simulink model "PLANTA_COMPLETA"  (R2024b)
settings: Solver=FixedStepAuto  StartTime=0.0  StopTime=inf  FixedStep=0.001  MaxStep=0.0005  RelTol=1e-4
undefined symbols (not defined in the file): A_hm, A_tm, at_breakpoints, at_max, b_ha, B_hm, b_ta, B_tm, bcx, bcy, bhd, bhEb, bhm, bt, btd, btm, btw, bwu, C_hm, C_tm, D_hm, D_tm, DiscIntNeverNeededParam, dl_h_ini, dx_l_ini, dx_t_ini, dx_td_ini, dxt_max, dy_l_ini, F01_a_t_max, F01_Ts1, F02_a_h_max, F02_Ts1, F03_a_h_max, F03_a_t_max, F03_dxt_max, F03_Ts1, Fhw_min, g, Hc, ih, it, Jhd_hEb, Jhm_hb, Jtd, Jtm_tb, K_hsa, K_hsia, K_tsa, K_tsia, Kcy, Kd_table, Ke_tita, Ke_w, kp_pos, Kp_table, kp_w, Ktw, kwu, l_breakpoints ... (+30)
libraries: simulink x13, spsEdgeDetectorLib x5, simulink_extras x2, dspsigops x2, vrlib x1, dspstat3 x1
(part 3 of 5)

== system PLANTA_COMPLETA/Masa contenedor ==
  Fwh : Inport
  TLK : Inport  Port=2
  Edge Detector : spsEdgeDetectorLib/Edge Detector  model=Falling  ic=0  Ts=-1
      settings: LibrarySourceBlock=sps_lib/Control/Edge Detector
  Edge Detector1 : spsEdgeDetectorLib/Edge Detector  model=Rising  ic=0  Ts=-1
      settings: LibrarySourceBlock=sps_lib/Control/Edge Detector
  Gain8 : Gain  Gain=2/g
  Product : Product
  S-R Flip-Flop : simulink_extras/Flip Flops/S-R Flip-Flop  initial_condition=0
  Unit Delay : UnitDelay  SampleTime=-1  HasFrameUpgradeWarning=on
  Mc_X : Outport
  wires:
  TLK/1 -> Unit Delay/1
  Edge Detector/1 -> S-R Flip-Flop/2
  Edge Detector1/1 -> S-R Flip-Flop/1
  S-R Flip-Flop/1 -> Product/2
  Product/1 -> Mc_X/1
  Unit Delay/1 -> Edge Detector1/1, Edge Detector/1
  Fwh/1 -> Gain8/1  "m estimada"
  Gain8/1 -> Product/1  "m estimada"

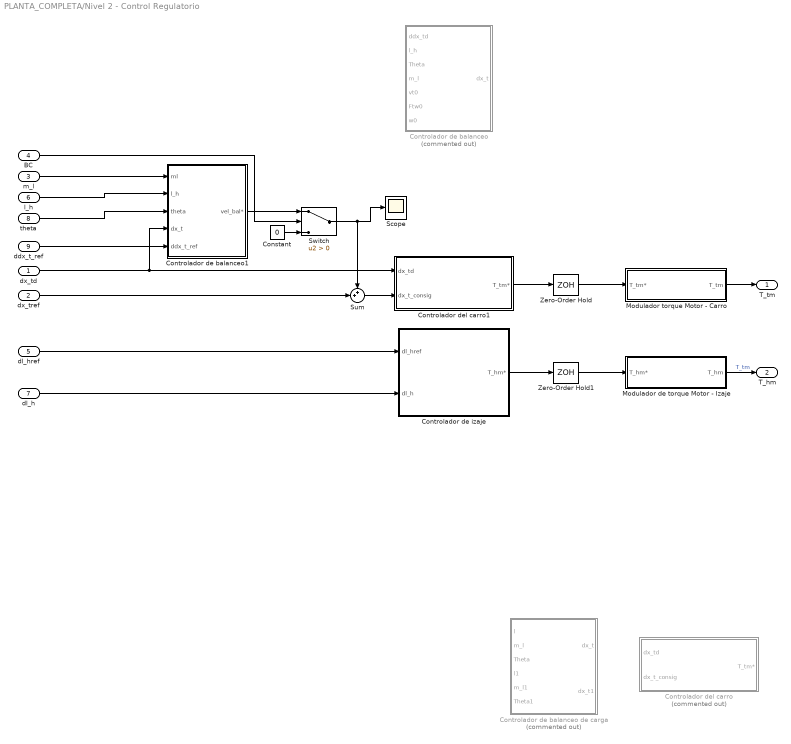
== system PLANTA_COMPLETA/Nivel 2 - Control Regulatorio ==
  dx_td : Inport
  dx_tref : Inport  Port=2
  m_l : Inport  Port=3
  BC : Inport  Port=4
  dl_href : Inport  Port=5
  l_h : Inport  Port=6
  dl_h : Inport  Port=7
  theta : Inport  Port=8
  ddx_t_ref : Inport  Port=9
  Constant : Constant  Value=0
  Controlador de balanceo : Subsystem  Commented=on
  Controlador de balanceo de carga : Subsystem  Commented=on
  Controlador de balanceo1 : Subsystem
  Controlador de izaje : Subsystem
  Controlador del carro : Subsystem  Commented=on
  Controlador del carro1 : Subsystem
  Modulador de torque Motor - Izaje : Subsystem
  Modulador torque Motor - Carro : Subsystem
  Scope : Scope
  Sum : Sum  Inputs=++|
  Switch : Switch  Criteria=u2 > Threshold  SaturateOnIntegerOverflow=off  InputSameDT=off
  Zero-Order Hold : ZeroOrderHold  SampleTime=T_s2
  Zero-Order Hold1 : ZeroOrderHold  SampleTime=T_s2
  T_tm : Outport
  T_hm : Outport  Port=2
  wires:
  dl_href/1 -> Controlador de izaje/1(dl_href)
  Zero-Order Hold1/1 -> Modulador de torque Motor - Izaje/1(T_hm*)
  dl_h/1 -> Controlador de izaje/2(dl_h)
  Controlador de izaje/1(T_hm*) -> Zero-Order Hold1/1
  Modulador de torque Motor - Izaje/1(T_hm) -> T_hm/1  "T_tm"
  Zero-Order Hold/1 -> Modulador torque Motor - Carro/1(T_tm*)
  Modulador torque Motor - Carro/1(T_tm) -> T_tm/1
  l_h/1 -> Controlador de balanceo1/2(l_h)
  dx_td/1 -> Controlador del carro1/1(dx_td), Controlador de balanceo1/4(dx_t)
  Constant/1 -> Switch/3
  m_l/1 -> Controlador de balanceo1/1(ml)
  BC/1 -> Switch/2
  Controlador del carro1/1(T_tm*) -> Zero-Order Hold/1
  Controlador de balanceo1/1(vel_bal*) -> Switch/1
  theta/1 -> Controlador de balanceo1/3(theta)
  dx_tref/1 -> Sum/2
  Sum/1 -> Controlador del carro1/2(dx_t_consig)
  Switch/1 -> Scope/1, Sum/1
  ddx_t_ref/1 -> Controlador de balanceo1/5(ddx_t_ref)

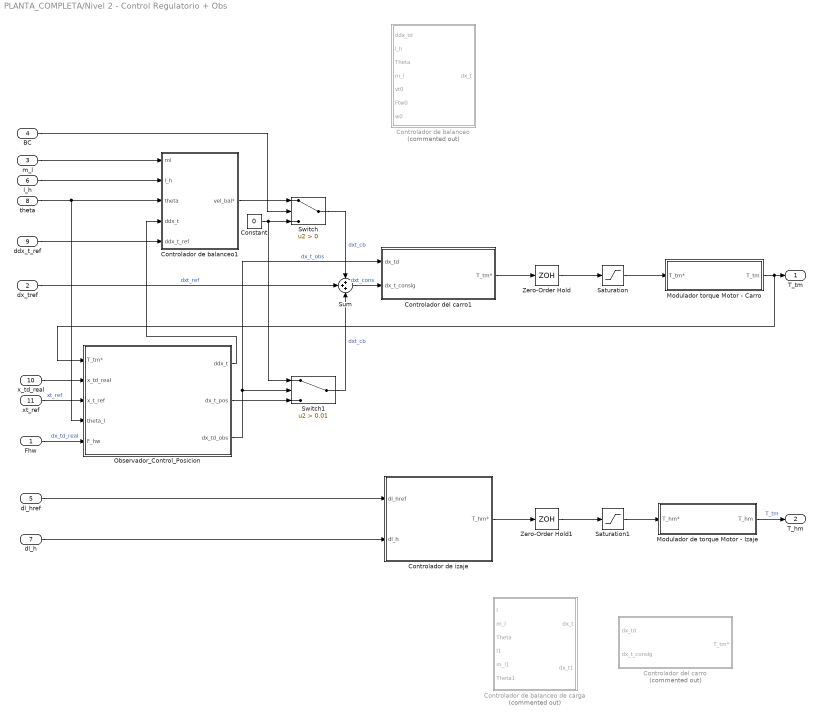
== system PLANTA_COMPLETA/Nivel 2 - Control Regulatorio + Obs ==
  Fhw : Inport
  dx_tref : Inport  Port=2
  m_l : Inport  Port=3
  BC : Inport  Port=4
  dl_href : Inport  Port=5
  l_h : Inport  Port=6
  dl_h : Inport  Port=7
  theta : Inport  Port=8
  ddx_t_ref : Inport  Port=9
  x_td_real : Inport  Port=10
  xt_ref : Inport  Port=11
  Constant : Constant  Value=0
  Controlador de balanceo : Subsystem  Commented=on
  Controlador de balanceo de carga : Subsystem  Commented=on
  Controlador de balanceo1 : Subsystem
  Controlador de izaje : Subsystem
  Controlador del carro : Subsystem  Commented=on
  Controlador del carro1 : Subsystem
  Modulador de torque Motor - Izaje : Subsystem
  Modulador torque Motor - Carro : Subsystem
  Observador_Control_Posicion : Subsystem
  Saturation : Saturate  UpperLimit=Ttm_Max  LowerLimit=-Ttm_Max
  Saturation1 : Saturate  UpperLimit=Thm_Max  LowerLimit=-Thm_Max
  Sum : Sum  Inputs=+++
  Switch : Switch  Criteria=u2 > Threshold  SaturateOnIntegerOverflow=off  InputSameDT=off
  Switch1 : Switch  Criteria=u2 > Threshold  Threshold=0.01  SaturateOnIntegerOverflow=off  InputSameDT=off
  Zero-Order Hold : ZeroOrderHold  SampleTime=T_s2
  Zero-Order Hold1 : ZeroOrderHold  SampleTime=T_s2
  T_tm : Outport
  T_hm : Outport  Port=2
  wires:
  dl_href/1 -> Controlador de izaje/1(dl_href)
  Zero-Order Hold1/1 -> Saturation1/1
  Controlador de izaje/1(T_hm*) -> Zero-Order Hold1/1
  Modulador de torque Motor - Izaje/1(T_hm) -> T_hm/1  "T_tm"
  Zero-Order Hold/1 -> Saturation/1
  Modulador torque Motor - Carro/1(T_tm) -> Observador_Control_Posicion/1(T_tm*), T_tm/1
  l_h/1 -> Controlador de balanceo1/2(l_h)
  Constant/1 -> Switch1/1, Switch/3
  m_l/1 -> Controlador de balanceo1/1(ml)
  BC/1 -> Switch/2
  Controlador del carro1/1(T_tm*) -> Zero-Order Hold/1
  Controlador de balanceo1/1(vel_bal*) -> Switch/1
  theta/1 -> Observador_Control_Posicion/4(theta_l), Controlador de balanceo1/3(theta)
  dx_tref/1 -> Sum/2  "dxt_ref"
  Sum/1 -> Controlador del carro1/2(dx_t_consig)  "dxt_cons"
  Switch/1 -> Sum/1  "dxt_cb"
  ddx_t_ref/1 -> Controlador de balanceo1/5(ddx_t_ref)
  Observador_Control_Posicion/3(dx_td_obs) -> Controlador del carro1/1(dx_td), Switch1/2  "dx_t_obs"
  Observador_Control_Posicion/1(ddx_t) -> Controlador de balanceo1/4(ddx_t)
  Observador_Control_Posicion/2(dx_t_pos) -> Switch1/3
  Switch1/1 -> Sum/3  "dxt_cb"
  xt_ref/1 -> Observador_Control_Posicion/3(x_t_ref)  "xt_ref"
  x_td_real/1 -> Observador_Control_Posicion/2(x_td_real)
  Fhw/1 -> Observador_Control_Posicion/5(F_hw)  "dx_td_real"
  dl_h/1 -> Controlador de izaje/2(dl_h)
  Saturation/1 -> Modulador torque Motor - Carro/1(T_tm*)
  Saturation1/1 -> Modulador de torque Motor - Izaje/1(T_hm*)

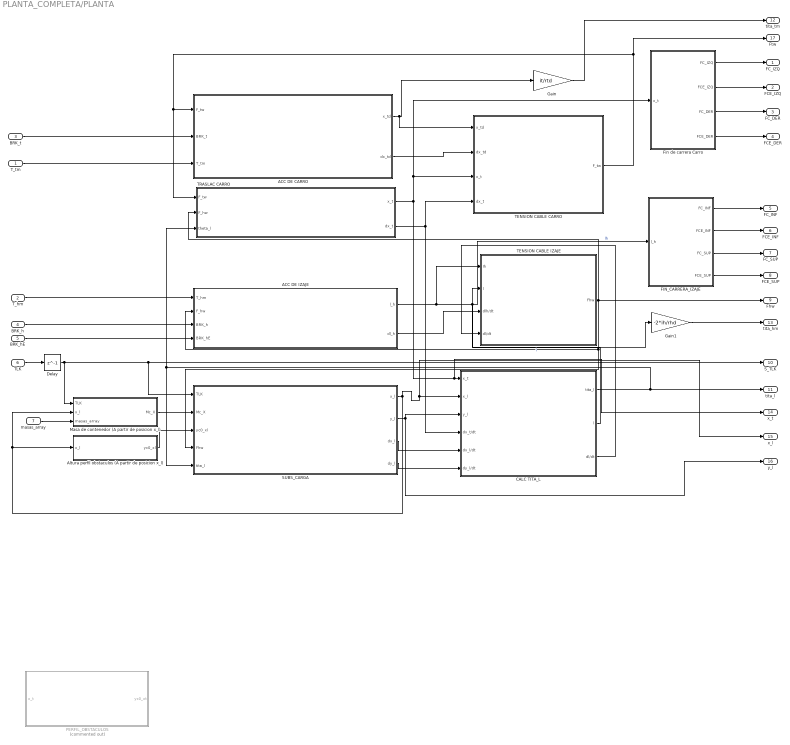
== system PLANTA_COMPLETA/PLANTA ==
  T_tm : Inport
  T_hm : Inport  Port=2
  BRK_t : Inport  Port=3
  BRK_h : Inport  Port=4
  BRK_hE : Inport  Port=5
  TLK : Inport  Port=6
  masas_array : Inport  Port=7
  ACC DE CARRO : Subsystem
  ACC DE IZAJE : Subsystem
  Altura perfil obstaculos (A partir de posicion x_l) : Subsystem
  CALC TITA_L : Subsystem
  Delay : Delay  DelayLength=1  InputProcessing=Columns as channels (frame based)  SampleTime=T_s1
  FIN_CARRERA_IZAJE : Subsystem
  Fin de carrera Carro : Subsystem
  Gain : Gain  Gain=it/rtd
  Gain1 : Gain  Gain=-2*ih/rhd
  Masa de contenedor (A partir de posicion x_l) : Subsystem
  PERFIL_OBSTACULOS : Subsystem  Commented=on
  SUBS_CARGA : Subsystem
  TENSION CABLE CARRO : Subsystem
  TENSION CABLE IZAJE : Subsystem
  TRASLAC CARRO : Subsystem
  FC_IZQ : Outport
  FCE_IZQ : Outport  Port=2
  FC_DER : Outport  Port=3
  FCE_DER : Outport  Port=4
  FC_INF : Outport  Port=5
  FCE_INF : Outport  Port=6
  FC_SUP : Outport  Port=7
  FCE_SUP : Outport  Port=8
  Fhw : Outport  Port=9
  S_TLK : Outport  Port=10
  tita_l : Outport  Port=11
  tita_tm : Outport  Port=12
  tita_hm : Outport  Port=13
  x_t : Outport  Port=14
  x_l : Outport  Port=15
  y_l : Outport  Port=16
  Ftw : Outport  Port=17
  wires:
  Gain/1 -> tita_tm/1
  TRASLAC CARRO/2(dx_t) -> TENSION CABLE CARRO/4(dx_t), CALC TITA_L/4(dx_t/dt)
  CALC TITA_L/3(dl/dt) -> TENSION CABLE IZAJE/4(dl/dt)
  BRK_h/1 -> ACC DE IZAJE/3(BRK_h)
  TLK/1 -> Delay/1
  BRK_t/1 -> ACC DE CARRO/2(BRK_t)
  ACC DE CARRO/1(x_td) -> Gain/1, TENSION CABLE CARRO/1(x_td)
  BRK_hE/1 -> ACC DE IZAJE/4(BRK_hE)
  ACC DE CARRO/2(dx_td) -> TENSION CABLE CARRO/2(dx_td)
  FIN_CARRERA_IZAJE/3(FC_SUP) -> FC_SUP/1
  Fin de carrera Carro/4(FCE_DER) -> FCE_DER/1
  SUBS_CARGA/4(dy_l) -> CALC TITA_L/6(dy_l/dt)
  TENSION CABLE CARRO/1(F_tw) -> Ftw/1, ACC DE CARRO/1(F_tw), TRASLAC CARRO/1(F_tw)
  SUBS_CARGA/3(dx_l) -> CALC TITA_L/5(dx_l/dt)
  Altura perfil obstaculos (A partir de posicion x_l)/1(yc0_xl) -> SUBS_CARGA/3(yc0_xl)
  ACC DE IZAJE/2(dl_h) -> TENSION CABLE IZAJE/3(dlh/dt)
  T_tm/1 -> ACC DE CARRO/3(T_tm)
  Fin de carrera Carro/2(FCE_IZQ) -> FCE_IZQ/1
  T_hm/1 -> ACC DE IZAJE/1(T_hm)
  FIN_CARRERA_IZAJE/1(FC_INF) -> FC_INF/1
  Gain1/1 -> tita_hm/1
  FIN_CARRERA_IZAJE/2(FCE_INF) -> FCE_INF/1
  Fin de carrera Carro/1(FC_IZQ) -> FC_IZQ/1
  FIN_CARRERA_IZAJE/4(FCE_SUP) -> FCE_SUP/1
  Fin de carrera Carro/3(FC_DER) -> FC_DER/1
  SUBS_CARGA/1(x_l) -> x_l/1, CALC TITA_L/2(x_l), Masa de contenedor (A partir de posicion x_l)/2(x_l), Altura perfil obstaculos (A partir de posicion x_l)/1(x_l)
  CALC TITA_L/1(tita_l) -> tita_l/1, TRASLAC CARRO/3(theta_l), SUBS_CARGA/5(tita_l)
  TRASLAC CARRO/1(x_t) -> Fin de carrera Carro/1(x_t), TENSION CABLE CARRO/3(x_t), CALC TITA_L/1(x_t), x_t/1
  SUBS_CARGA/2(y_l) -> y_l/1, CALC TITA_L/3(y_l)
  Masa de contenedor (A partir de posicion x_l)/1(Mc_X) -> SUBS_CARGA/2(Mc_X)
  Delay/1 -> Masa de contenedor (A partir de posicion x_l)/1(TLK), S_TLK/1, SUBS_CARGA/1(TLK)
  masas_array/1 -> Masa de contenedor (A partir de posicion x_l)/3(masas_array)
  ACC DE IZAJE/1(l_h) -> Gain1/1, FIN_CARRERA_IZAJE/1(l_h), TENSION CABLE IZAJE/1(Ih)  "lh"
  CALC TITA_L/2(l) -> TENSION CABLE IZAJE/2(l)  "l"
  TENSION CABLE IZAJE/1(Fhw) -> SUBS_CARGA/4(Fhw), ACC DE IZAJE/2(F_hw), TRASLAC CARRO/2(F_hw), Fhw/1

== system PLANTA_COMPLETA/Actualizar perfil/Enabled Subsystem ==
  index : Inport
  Enable : EnablePort
  Actualiza perfil : MATLAB Function  TreatAsAtomicUnit=on
  Constant16 : Constant  Value=Hc
  Data Store Read3 : DataStoreRead  DataStoreName=y0_global  IndexOptions=Index vector (dialog)  Indices=1  OutputSizes=1
  y0_actualizado : Outport
  wires:
  Data Store Read3/1 -> Actualiza perfil/2(y0)
  Constant16/1 -> Actualiza perfil/3(Hc)
  index/1 -> Actualiza perfil/1(index)
  Actualiza perfil/1(y0_actualizado) -> y0_actualizado/1

== system PLANTA_COMPLETA/Nivel 2 - Control Regulatorio/Controlador de balanceo ==
  note: Controlador
  ddx_td : Inport
  l_h : Inport  Port=2
  Theta : Inport  Port=3
  m_l : Inport  Port=4
  vt0 : Inport  Port=5
  Ftw0 : Inport  Port=6
  w0 : Inport  Port=7
  Atan : Trigonometry  Operator=atan
  Constant1 : Constant  Value=Mt
  Constant3 : Constant  Value=bt
  Constant4 : Constant  Value=g
  Constant5 : Constant  Value=0
  Discrete Derivative1 : simulink/Discrete/Discrete Derivative  gainval=1.0  ICPrevScaledInput=0.0  OutMin=[]  OutMax=[]  OutDataType=fixdt(1, 16)  OutScaling=2^-10  DoSatur=off
  Gain : Gain  Gain=1/g
  MATLAB Function : MATLAB Function  TreatAsAtomicUnit=on
  Product1 : Product
  Product7 : Product
  Sum1 : Sum  Inputs=|-+
  Sum11 : Sum  Inputs=|++
  dx_t : Outport
  wires:
  Discrete Derivative1/1 -> Product7/1
  Sum11/1 -> dx_t/1
  MATLAB Function/2(Kd) -> Product7/2  "Kd"
  Product7/1 -> Sum11/2
  Constant1/1 -> MATLAB Function/6(Mt0)
  m_l/1 -> MATLAB Function/7(ml0)
  Constant3/1 -> MATLAB Function/9(bt0)
  Constant4/1 -> MATLAB Function/10(g0)
  Constant5/1 -> MATLAB Function/1(xt0)
  vt0/1 -> MATLAB Function/2(vt0)
  w0/1 -> MATLAB Function/4(w0)
  ddx_td/1 -> Gain/1
  Gain/1 -> Atan/1
  l_h/1 -> MATLAB Function/8(l0)
  Atan/1 -> Sum1/2
  MATLAB Function/1(Kp) -> Product1/1  "Kp"
  Sum1/1 -> Discrete Derivative1/1, Product1/2
  Ftw0/1 -> MATLAB Function/5(Ftw0)
  Theta/1 -> Sum1/1, MATLAB Function/3(th0)
  Product1/1 -> Sum11/1

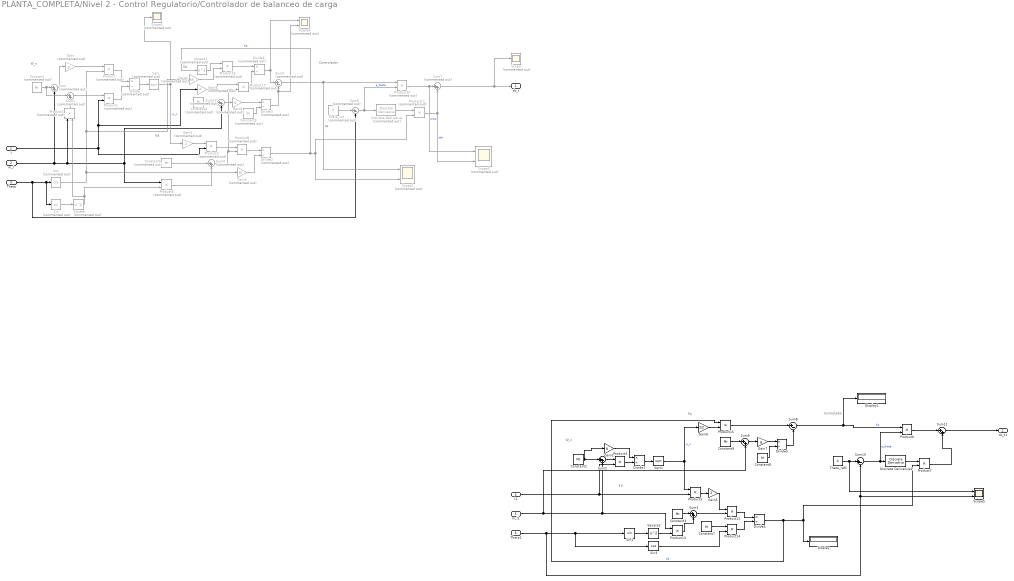
== system PLANTA_COMPLETA/Nivel 2 - Control Regulatorio/Controlador de balanceo de carga ==
  note: Kp
  note: W_n
  note: Controlador
  note: Kd
  note: W_n
  note: Controlador
  note: Kp
  note: Kd
  l : Inport
  m_l : Inport  Port=2
  Theta : Inport  Port=3
  l1 : Inport  Port=4
  m_l1 : Inport  Port=5
  Theta1 : Inport  Port=6
  Constant : Constant  Commented=on  Value=Mt
  Constant1 : Constant  Commented=on  Value=Mt
  Constant2 : Constant  Value=Mt
  Constant3 : Constant  Value=Mt
  Constant4 : Constant  Commented=on  Value=Mt
  Constant5 : Constant  Commented=on  Value=bt
  Constant7 : Constant  Value=bt
  Constant8 : Constant  Value=bt
  Constant9 : Constant  Value=Mt
  Cos : Trigonometry  Commented=on  Operator=cos
  Discrete Derivative : simulink/Discrete/Discrete Derivative  Commented=on  gainval=1/T_s2  ICPrevScaledInput=0.0  OutMin=[]  OutMax=[]  OutDataType=fixdt(1, 16)  OutScaling=2^-10  DoSatur=off
  Discrete Derivative1 : simulink/Discrete/Discrete Derivative  gainval=1.0  ICPrevScaledInput=0.0  OutMin=[]  OutMax=[]  OutDataType=fixdt(1, 16)  OutScaling=2^-10  DoSatur=off
  Display : Display
  Display1 : Display
  Divide{,2..3,6} (4 alike) : Product  Commented=on  Inputs=*/
  Divide1 : Product  Inputs=*/
  Divide4 : Product  Inputs=*/
  Divide5 : Product  Inputs=*/
  Gain : Gain  Commented=on  Gain=g
  Gain1 : Gain  Gain=g
  Gain2 : Gain  Commented=on  Gain=2
  Gain3 : Gain  Commented=on  Gain=bt
  Gain4 : Gain  Commented=on  Gain=bt
  Gain5 : Gain  Gain=2
  Gain6 : Gain  Gain=1/2
  Gain7 : Gain  Gain=g
  Gain8 : Gain  Commented=on  Gain=g
  Gain9 : Gain  Commented=on  Gain=4
  Product{,1..3,8..11,16..17} (10 alike) : Product  Commented=on
  Product{4..7,12..15} (8 alike) : Product
  Scope : Scope  Commented=on
  Scope1 : Scope  Commented=on  NumInputPorts=2
  Scope2 : Scope  Commented=on
  Scope3 : Scope  Commented=on  NumInputPorts=2
  Scope4 : Scope  Commented=on  NumInputPorts=2
  Scope5 : Scope  NumInputPorts=2
  Sin : Trigonometry  Commented=on
  Sin1 : Trigonometry
  Sin3 : Trigonometry  Operator=cos
  Sqrt : Sqrt  Commented=on
  Sqrt1 : Sqrt
  Square : Math  Commented=on  Operator=square
  Square1 : Math  Commented=on  Operator=square
  Square2 : Math  Operator=square
  Sum{,1,4,7,12} (5 alike) : Sum  Commented=on  Inputs=|++
  Sum10 : Sum  Inputs=|+-
  Sum{2..3,9,11} (4 alike) : Sum  Inputs=|++
  Sum5 : Sum  Commented=on  Inputs=|+-
  Sum6 : Sum  Commented=on  Inputs=|+-
  Sum8 : Sum  Inputs=|+-
  Theta_ref : Constant  Commented=on  Value=0
  Theta_ref1 : Constant  Value=0
  dx_t : Outport
  dx_t1 : Outport  Port=2
  wires:
  Theta_ref/1 -> Sum6/1
  Sum6/1 -> Product10/2, Discrete Derivative/1  "e_theta"
  Product11/1 -> Scope3/2, Sum7/2  "der"
  Divide/1 -> Sqrt/1
  Sum/1 -> Gain/1
  Theta/1 -> Sin/1, Cos/1, Sum6/2
  m_l/1 -> Sum/2, Product8/1, Sum12/2, Product2/1
  Product10/1 -> Scope3/1, Sum7/1  "prop"
  Product/1 -> Divide/1
  Product15/1 -> Sum8/1
  Gain1/1 -> Divide1/1
  Constant3/1 -> Sum3/1
  Product14/1 -> Divide4/2
  Sin3/1 -> Product14/2
  Product4/1 -> Divide1/2
  Divide5/1 -> Sum8/2
  Sum8/1 -> Display1/1, Product6/1  "Kp"
  Constant9/1 -> Sum9/1
  Sqrt1/1 -> Product5/1, Gain6/1  "w_n"
  Sum2/1 -> Product4/1
  Theta_ref1/1 -> Scope5/1, Sum10/1
  Sin1/1 -> Square2/1
  Sum11/1 -> dx_t1/1
  Constant8/1 -> Divide5/2
  Sum9/1 -> Gain7/1
  Constant2/1 -> Gain1/1, Sum2/1
  Constant7/1 -> Product14/1
  Product5/1 -> Gain5/1
  Theta1/1 -> Sin3/1, Sin1/1, Scope5/2, Sum10/2
  l1/1 -> Product4/2, Product5/2
  Gain7/1 -> Divide5/1
  Sum10/1 -> Product6/2, Discrete Derivative1/1  "e_theta"
  Gain6/1 -> Product15/2
  Divide4/1 -> Product7/2, Display/1, Product15/1  "Kd"
  Discrete Derivative1/1 -> Product7/1
  Gain5/1 -> Product12/1
  Square2/1 -> Product13/2
  Product12/1 -> Divide4/1
  m_l1/1 -> Product13/1, Sum2/2, Sum9/2
  Product7/1 -> Sum11/2
  Product13/1 -> Sum3/2
  Sum3/1 -> Product12/2
  Product6/1 -> Sum11/1
  Divide1/1 -> Sqrt1/1
  Constant/1 -> Sum1/1, Sum/1
  Sin/1 -> Square/1
  Cos/1 -> Gain4/1, Product/2, Gain3/1
  Gain/1 -> Product/1
  l/1 -> Gain9/1, Product1/2, Product3/2
  Sum1/1 -> Product1/1
  Product2/1 -> Sum1/2
  Square/1 -> Product8/2, Product2/2
  Product1/1 -> Divide/2
  Sqrt/1 -> Scope2/1, Gain2/1  "w_n"
  Gain2/1 -> Product3/1
  Constant1/1 -> Sum4/1
  Product8/1 -> Sum4/2
  Sum4/1 -> Product9/2, Product17/2
  Product3/1 -> Product9/1
  Product9/1 -> Divide2/1
  Gain3/1 -> Divide2/2
  Divide2/1 -> Square1/1, Product11/2, Scope1/2  "Kd"
  Constant4/1 -> Sum12/1
  Sum12/1 -> Gain8/1
  Gain8/1 -> Divide3/1
  Divide3/1 -> Scope4/2, Sum5/2
  Sum5/1 -> Scope1/1, Product10/1  "Kp"
  Sum7/1 -> dx_t/1, Scope/1
  Constant5/1 -> Divide3/2
  Discrete Derivative/1 -> Product11/1
  Gain4/1 -> Product16/2
  Square1/1 -> Product16/1
  Product16/1 -> Divide6/1
  Gain9/1 -> Product17/1
  Product17/1 -> Divide6/2
  Divide6/1 -> Scope4/1, Sum5/1

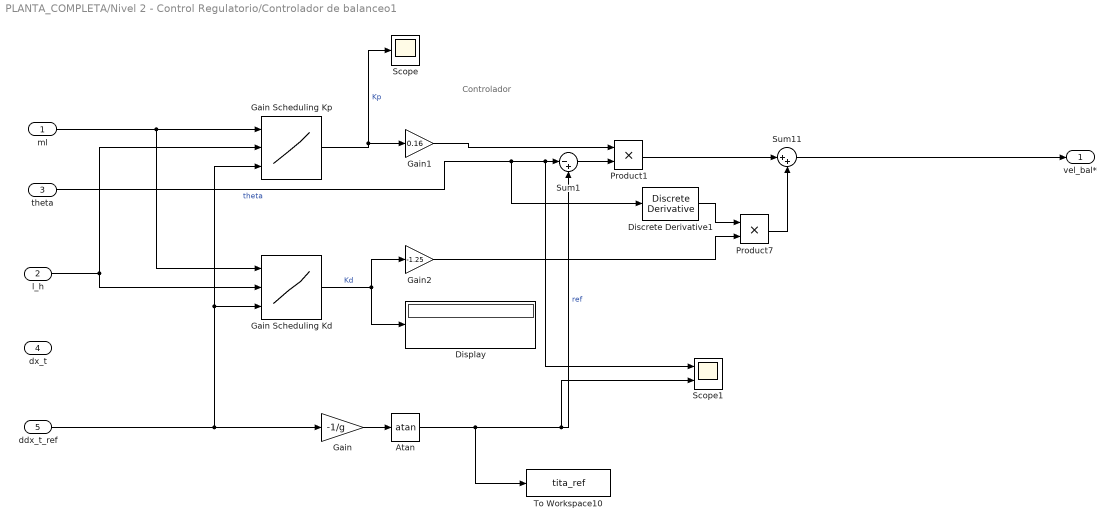
== system PLANTA_COMPLETA/Nivel 2 - Control Regulatorio/Controlador de balanceo1 ==
  note: Controlador
  ml : Inport
  l_h : Inport  Port=2
  theta : Inport  Port=3
  dx_t : Inport  Port=4
  ddx_t_ref : Inport  Port=5
  Atan : Trigonometry  Operator=atan
  Discrete Derivative1 : simulink/Discrete/Discrete Derivative  gainval=1.0  ICPrevScaledInput=0.0  OutMin=[]  OutMax=[]  OutDataType=fixdt(1, 16)  OutScaling=2^-10  DoSatur=off
  Display : Display
  Gain : Gain  Gain=-1/g
  Gain Scheduling Kd : Lookup_n-D  NumberOfTableDimensions=3  BreakpointsForDimension1=ml_breakpoints  BreakpointsForDimension2=l_breakpoints  BreakpointsForDimension3=at_breakpoints  BreakpointsForDimension4=at_breakpoints  Table=Kd_table  InterpMethod=Flat  ExtrapMethod=Clip  InternalRulePriority=Speed  RndMeth=Simplest
      settings: InputPortMap=u0,u1,u2
  Gain Scheduling Kp : Lookup_n-D  NumberOfTableDimensions=3  BreakpointsForDimension1=ml_breakpoints  BreakpointsForDimension2=l_breakpoints  BreakpointsForDimension3=at_breakpoints  BreakpointsForDimension4=at_breakpoints  Table=Kp_table  InterpMethod=Flat  ExtrapMethod=Clip  InternalRulePriority=Speed  RndMeth=Simplest
      settings: InputPortMap=u0,u1,u2
  Gain1 : Gain  Gain=0.16
  Gain2 : Gain  Gain=-1.25
  Product1 : Product
  Product7 : Product
  Scope : Scope
  Scope1 : Scope  NumInputPorts=2
  Sum1 : Sum  Inputs=|-+
  Sum11 : Sum  Inputs=|++
  To Workspace10 : ToWorkspace  VariableName=tita_ref  SaveFormat=Timeseries  SampleTime=-1
      settings: Save2DSignal=2-D array (concatenate along first dimension)
  vel_bal* : Outport
  wires:
  Discrete Derivative1/1 -> Product7/1
  Gain Scheduling Kd/1 -> Gain2/1, Display/1  "Kd"
  Gain/1 -> Atan/1
  Gain Scheduling Kp/1 -> Scope/1, Gain1/1  "Kp"
  l_h/1 -> Gain Scheduling Kd/2, Gain Scheduling Kp/2
  theta/1 -> Discrete Derivative1/1, Scope1/1, Sum1/1  "theta"
  Sum1/1 -> Product1/2
  Product1/1 -> Sum11/1
  Atan/1 -> To Workspace10/1, Scope1/2, Sum1/2  "ref"
  Sum11/1 -> vel_bal*/1
  Product7/1 -> Sum11/2
  ddx_t_ref/1 -> Gain Scheduling Kp/3, Gain Scheduling Kd/3, Gain/1
  ml/1 -> Gain Scheduling Kd/1, Gain Scheduling Kp/1
  Gain1/1 -> Product1/1
  Gain2/1 -> Product7/2

== system PLANTA_COMPLETA/Nivel 2 - Control Regulatorio/Controlador de izaje ==
  dl_href : Inport
  dl_h : Inport  Port=2
  Gain : Gain  Gain=T_s2/2
  Gain1 : Gain  Gain=K_hsia
  Gain2 : Gain  Gain=b_ha
  Gain3 : Gain  Gain=T_s2/2
  Gain8 : Gain  Gain=K_hsa
  Sum : Sum  Inputs=|+-
  Sum{1..4} (4 alike) : Sum  Inputs=|++
  Sum5 : Sum  Inputs=+|+|+
  Unit Delay{,1..3} (4 alike) : UnitDelay  SampleTime=-1  HasFrameUpgradeWarning=on
  T_hm* : Outport
  wires:
  Gain2/1 -> Sum5/3
  Unit Delay1/1 -> Sum2/2  "Ik-1"
  Unit Delay3/1 -> Sum4/2  "Ik-1"
  dl_h/1 -> Sum/2
  Unit Delay/1 -> Sum1/2  "d_ek-1"
  Gain/1 -> Sum2/1  "Ik"
  Gain3/1 -> Sum4/1  "Ik"
  Sum5/1 -> T_hm*/1
  dl_href/1 -> Sum/1
  Gain1/1 -> Sum5/1
  Sum/1 -> Gain2/1, Unit Delay/1, Sum1/1  "d_ek"
  Sum4/1 -> Unit Delay3/1, Gain1/1
  Unit Delay2/1 -> Sum3/2  "ek-1"
  Sum3/1 -> Gain3/1
  Sum2/1 -> Sum3/1, Unit Delay2/1, Gain8/1, Unit Delay1/1  "ek"
  Gain8/1 -> Sum5/2
  Sum1/1 -> Gain/1

== system PLANTA_COMPLETA/Nivel 2 - Control Regulatorio/Controlador del carro ==
  dx_td : Inport
  dx_t_consig : Inport  Port=2
  Gain : Gain  Gain=T_s2/2
  Gain1 : Gain  Gain=b_ta
  Gain2 : Gain  Gain=K_tsa
  Gain3 : Gain  Gain=T_s2/2
  Gain4 : Gain  Gain=K_tsia
  Scope : Scope
  Scope1 : Scope
  Sum : Sum  Inputs=|+-
  Sum1 : Sum  Inputs=|+-
  Sum2 : Sum  Inputs=|++
  Sum3 : Sum  Inputs=|+-
  Sum4 : Sum  Inputs=|++
  Sum5 : Sum  Inputs=+|+|+
  Unit Delay{,1..3} (4 alike) : UnitDelay  SampleTime=T_s2  HasFrameUpgradeWarning=on
  T_tm* : Outport
  wires:
  Unit Delay3/1 -> Sum4/2  "Ik-1"
  Unit Delay2/1 -> Sum3/2  "ek-1"
  Sum/1 -> Gain1/1, Unit Delay/1, Sum1/1  "d_ek"
  dx_t_consig/1 -> Sum/1
  Gain3/1 -> Sum4/1  "Ik"
  Sum5/1 -> T_tm*/1
  dx_td/1 -> Sum/2
  Sum1/1 -> Gain/1
  Unit Delay/1 -> Sum1/2  "d_ek-1"
  Sum2/1 -> Unit Delay1/1, Sum3/1, Unit Delay2/1, Scope/1, Gain2/1  "ek"
  Gain/1 -> Sum2/1  "Ik"
  Gain2/1 -> Sum5/2
  Sum3/1 -> Gain3/1
  Unit Delay1/1 -> Sum2/2  "Ik-1"
  Sum4/1 -> Gain4/1, Unit Delay3/1
  Gain1/1 -> Sum5/3
  Gain4/1 -> Scope1/1, Sum5/1

== system PLANTA_COMPLETA/Nivel 2 - Control Regulatorio/Controlador del carro1 ==
  dx_td : Inport
  dx_t_consig : Inport  Port=2
  Gain : Gain  Gain=T_s2/2
  Gain1 : Gain  Gain=b_ta
  Gain2 : Gain  Gain=K_tsa
  Gain3 : Gain  Gain=T_s2/2
  Gain4 : Gain  Gain=K_tsia
  Scope : Scope
  Scope1 : Scope
  Sum : Sum  Inputs=|+-
  Sum1 : Sum  Inputs=|+-
  Sum2 : Sum  Inputs=|++
  Sum3 : Sum  Inputs=|+-
  Sum4 : Sum  Inputs=|++
  Sum5 : Sum  Inputs=+|+|+
  Unit Delay{,1..3} (4 alike) : UnitDelay  SampleTime=T_s2  HasFrameUpgradeWarning=on
  T_tm* : Outport
  wires:
  Unit Delay3/1 -> Sum4/2  "Ik-1"
  Unit Delay2/1 -> Sum3/2  "ek-1"
  Sum/1 -> Gain1/1, Unit Delay/1, Sum1/1  "d_ek"
  dx_t_consig/1 -> Sum/1
  Gain3/1 -> Sum4/1  "Ik"
  Sum5/1 -> T_tm*/1
  dx_td/1 -> Sum/2
  Sum1/1 -> Gain/1
  Unit Delay/1 -> Sum1/2  "d_ek-1"
  Sum2/1 -> Unit Delay1/1, Sum3/1, Unit Delay2/1, Scope/1, Gain2/1  "ek"
  Gain/1 -> Sum2/1  "Ik"
  Gain2/1 -> Sum5/2
  Sum3/1 -> Gain3/1
  Unit Delay1/1 -> Sum2/2  "Ik-1"
  Sum4/1 -> Gain4/1, Unit Delay3/1
  Gain1/1 -> Sum5/3
  Gain4/1 -> Scope1/1, Sum5/1

== system PLANTA_COMPLETA/Nivel 2 - Control Regulatorio/Modulador de torque Motor - Izaje ==
  T_hm* : Inport
  State-Space : StateSpace  A=A_hm  B=B_hm  C=C_hm  D=D_hm  InitialCondition=0
  T_hm : Outport
  wires:
  T_hm*/1 -> State-Space/1
  State-Space/1 -> T_hm/1

== system PLANTA_COMPLETA/Nivel 2 - Control Regulatorio/Modulador torque Motor - Carro ==
  T_tm* : Inport
  State-Space : StateSpace  A=A_tm  B=B_tm  C=C_tm  D=D_tm  InitialCondition=0
  T_tm : Outport
  wires:
  State-Space/1 -> T_tm/1
  T_tm*/1 -> State-Space/1

== system PLANTA_COMPLETA/Nivel 2 - Control Regulatorio + Obs/Controlador de balanceo ==
  note: Controlador
  ddx_td : Inport
  l_h : Inport  Port=2
  Theta : Inport  Port=3
  m_l : Inport  Port=4
  vt0 : Inport  Port=5
  Ftw0 : Inport  Port=6
  w0 : Inport  Port=7
  Atan : Trigonometry  Operator=atan
  Constant1 : Constant  Value=Mt
  Constant3 : Constant  Value=bt
  Constant4 : Constant  Value=g
  Constant5 : Constant  Value=0
  Discrete Derivative1 : simulink/Discrete/Discrete Derivative  gainval=1.0  ICPrevScaledInput=0.0  OutMin=[]  OutMax=[]  OutDataType=fixdt(1, 16)  OutScaling=2^-10  DoSatur=off
  Gain : Gain  Gain=1/g
  MATLAB Function : MATLAB Function  TreatAsAtomicUnit=on
  Product1 : Product
  Product7 : Product
  Sum1 : Sum  Inputs=|-+
  Sum11 : Sum  Inputs=|++
  dx_t : Outport
  wires:
  Discrete Derivative1/1 -> Product7/1
  Sum11/1 -> dx_t/1
  MATLAB Function/2(Kd) -> Product7/2  "Kd"
  Product7/1 -> Sum11/2
  Constant1/1 -> MATLAB Function/6(Mt0)
  m_l/1 -> MATLAB Function/7(ml0)
  Constant3/1 -> MATLAB Function/9(bt0)
  Constant4/1 -> MATLAB Function/10(g0)
  Constant5/1 -> MATLAB Function/1(xt0)
  vt0/1 -> MATLAB Function/2(vt0)
  w0/1 -> MATLAB Function/4(w0)
  ddx_td/1 -> Gain/1
  Gain/1 -> Atan/1
  l_h/1 -> MATLAB Function/8(l0)
  Atan/1 -> Sum1/2
  MATLAB Function/1(Kp) -> Product1/1  "Kp"
  Sum1/1 -> Discrete Derivative1/1, Product1/2
  Ftw0/1 -> MATLAB Function/5(Ftw0)
  Theta/1 -> Sum1/1, MATLAB Function/3(th0)
  Product1/1 -> Sum11/1

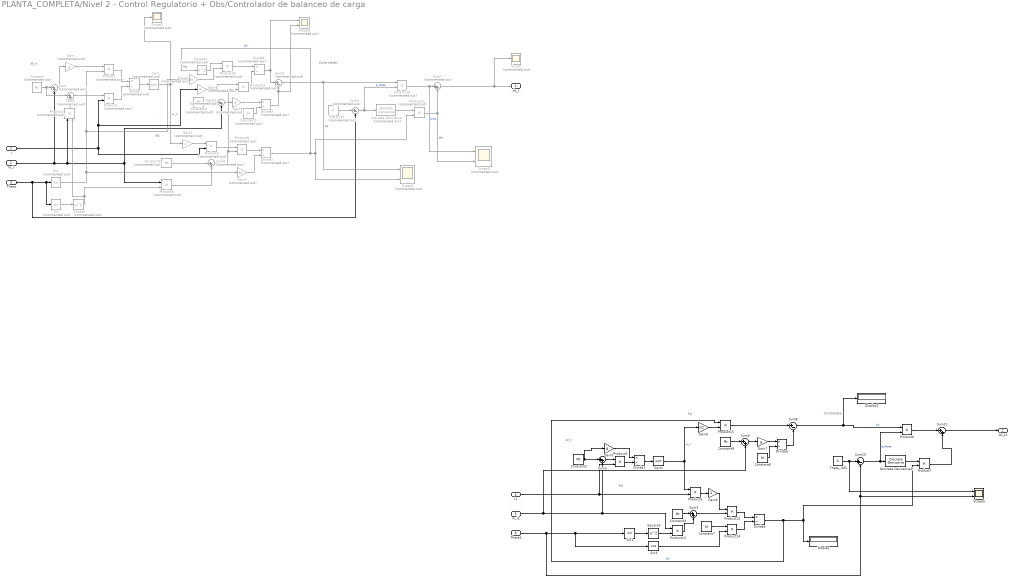
== system PLANTA_COMPLETA/Nivel 2 - Control Regulatorio + Obs/Controlador de balanceo de carga ==
  note: Kp
  note: W_n
  note: Controlador
  note: Kd
  note: W_n
  note: Controlador
  note: Kp
  note: Kd
  l : Inport
  m_l : Inport  Port=2
  Theta : Inport  Port=3
  l1 : Inport  Port=4
  m_l1 : Inport  Port=5
  Theta1 : Inport  Port=6
  Constant : Constant  Commented=on  Value=Mt
  Constant1 : Constant  Commented=on  Value=Mt
  Constant2 : Constant  Value=Mt
  Constant3 : Constant  Value=Mt
  Constant4 : Constant  Commented=on  Value=Mt
  Constant5 : Constant  Commented=on  Value=bt
  Constant7 : Constant  Value=bt
  Constant8 : Constant  Value=bt
  Constant9 : Constant  Value=Mt
  Cos : Trigonometry  Commented=on  Operator=cos
  Discrete Derivative : simulink/Discrete/Discrete Derivative  Commented=on  gainval=1/T_s2  ICPrevScaledInput=0.0  OutMin=[]  OutMax=[]  OutDataType=fixdt(1, 16)  OutScaling=2^-10  DoSatur=off
  Discrete Derivative1 : simulink/Discrete/Discrete Derivative  gainval=1.0  ICPrevScaledInput=0.0  OutMin=[]  OutMax=[]  OutDataType=fixdt(1, 16)  OutScaling=2^-10  DoSatur=off
  Display : Display
  Display1 : Display
  Divide{,2..3,6} (4 alike) : Product  Commented=on  Inputs=*/
  Divide1 : Product  Inputs=*/
  Divide4 : Product  Inputs=*/
  Divide5 : Product  Inputs=*/
  Gain : Gain  Commented=on  Gain=g
  Gain1 : Gain  Gain=g
  Gain2 : Gain  Commented=on  Gain=2
  Gain3 : Gain  Commented=on  Gain=bt
  Gain4 : Gain  Commented=on  Gain=bt
  Gain5 : Gain  Gain=2
  Gain6 : Gain  Gain=1/2
  Gain7 : Gain  Gain=g
  Gain8 : Gain  Commented=on  Gain=g
  Gain9 : Gain  Commented=on  Gain=4
  Product{,1..3,8..11,16..17} (10 alike) : Product  Commented=on
  Product{4..7,12..15} (8 alike) : Product
  Scope : Scope  Commented=on
  Scope1 : Scope  Commented=on  NumInputPorts=2
  Scope2 : Scope  Commented=on
  Scope3 : Scope  Commented=on  NumInputPorts=2
  Scope4 : Scope  Commented=on  NumInputPorts=2
  Scope5 : Scope  NumInputPorts=2
  Sin : Trigonometry  Commented=on
  Sin1 : Trigonometry
  Sin3 : Trigonometry  Operator=cos
  Sqrt : Sqrt  Commented=on
  Sqrt1 : Sqrt
  Square : Math  Commented=on  Operator=square
  Square1 : Math  Commented=on  Operator=square
  Square2 : Math  Operator=square
  Sum{,1,4,7,12} (5 alike) : Sum  Commented=on  Inputs=|++
  Sum10 : Sum  Inputs=|+-
  Sum{2..3,9,11} (4 alike) : Sum  Inputs=|++
  Sum5 : Sum  Commented=on  Inputs=|+-
  Sum6 : Sum  Commented=on  Inputs=|+-
  Sum8 : Sum  Inputs=|+-
  Theta_ref : Constant  Commented=on  Value=0
  Theta_ref1 : Constant  Value=0
  dx_t : Outport
  dx_t1 : Outport  Port=2
  wires:
  Theta_ref/1 -> Sum6/1
  Sum6/1 -> Product10/2, Discrete Derivative/1  "e_theta"
  Product11/1 -> Scope3/2, Sum7/2  "der"
  Divide/1 -> Sqrt/1
  Sum/1 -> Gain/1
  Theta/1 -> Sin/1, Cos/1, Sum6/2
  m_l/1 -> Sum/2, Product8/1, Sum12/2, Product2/1
  Product10/1 -> Scope3/1, Sum7/1  "prop"
  Product/1 -> Divide/1
  Product15/1 -> Sum8/1
  Gain1/1 -> Divide1/1
  Constant3/1 -> Sum3/1
  Product14/1 -> Divide4/2
  Sin3/1 -> Product14/2
  Product4/1 -> Divide1/2
  Divide5/1 -> Sum8/2
  Sum8/1 -> Display1/1, Product6/1  "Kp"
  Constant9/1 -> Sum9/1
  Sqrt1/1 -> Product5/1, Gain6/1  "w_n"
  Sum2/1 -> Product4/1
  Theta_ref1/1 -> Scope5/1, Sum10/1
  Sin1/1 -> Square2/1
  Sum11/1 -> dx_t1/1
  Constant8/1 -> Divide5/2
  Sum9/1 -> Gain7/1
  Constant2/1 -> Gain1/1, Sum2/1
  Constant7/1 -> Product14/1
  Product5/1 -> Gain5/1
  Theta1/1 -> Sin3/1, Sin1/1, Scope5/2, Sum10/2
  l1/1 -> Product4/2, Product5/2
  Gain7/1 -> Divide5/1
  Sum10/1 -> Product6/2, Discrete Derivative1/1  "e_theta"
  Gain6/1 -> Product15/2
  Divide4/1 -> Product7/2, Display/1, Product15/1  "Kd"
  Discrete Derivative1/1 -> Product7/1
  Gain5/1 -> Product12/1
  Square2/1 -> Product13/2
  Product12/1 -> Divide4/1
  m_l1/1 -> Product13/1, Sum2/2, Sum9/2
  Product7/1 -> Sum11/2
  Product13/1 -> Sum3/2
  Sum3/1 -> Product12/2
  Product6/1 -> Sum11/1
  Divide1/1 -> Sqrt1/1
  Constant/1 -> Sum1/1, Sum/1
  Sin/1 -> Square/1
  Cos/1 -> Gain4/1, Product/2, Gain3/1
  Gain/1 -> Product/1
  l/1 -> Gain9/1, Product1/2, Product3/2
  Sum1/1 -> Product1/1
  Product2/1 -> Sum1/2
  Square/1 -> Product8/2, Product2/2
  Product1/1 -> Divide/2
  Sqrt/1 -> Scope2/1, Gain2/1  "w_n"
  Gain2/1 -> Product3/1
  Constant1/1 -> Sum4/1
  Product8/1 -> Sum4/2
  Sum4/1 -> Product9/2, Product17/2
  Product3/1 -> Product9/1
  Product9/1 -> Divide2/1
  Gain3/1 -> Divide2/2
  Divide2/1 -> Square1/1, Product11/2, Scope1/2  "Kd"
  Constant4/1 -> Sum12/1
  Sum12/1 -> Gain8/1
  Gain8/1 -> Divide3/1
  Divide3/1 -> Scope4/2, Sum5/2
  Sum5/1 -> Scope1/1, Product10/1  "Kp"
  Sum7/1 -> dx_t/1, Scope/1
  Constant5/1 -> Divide3/2
  Discrete Derivative/1 -> Product11/1
  Gain4/1 -> Product16/2
  Square1/1 -> Product16/1
  Product16/1 -> Divide6/1
  Gain9/1 -> Product17/1
  Product17/1 -> Divide6/2
  Divide6/1 -> Scope4/1, Sum5/1

== system PLANTA_COMPLETA/Nivel 2 - Control Regulatorio + Obs/Controlador de balanceo1 ==
  note: Controlador
  ml : Inport
  l_h : Inport  Port=2
  theta : Inport  Port=3
  ddx_t : Inport  Port=4
  ddx_t_ref : Inport  Port=5
  Atan : Trigonometry  Operator=atan  ApproximationMethod=Lookup
  Delay : Delay  DelayLength=1  InputProcessing=Columns as channels (frame based)  SampleTime=T_s2
  Gain : Gain  Gain=-1/g
  Gain Scheduling Kd : Lookup_n-D  NumberOfTableDimensions=3  BreakpointsForDimension1=ml_breakpoints  BreakpointsForDimension2=l_breakpoints  BreakpointsForDimension3=at_breakpoints  BreakpointsForDimension4=at_breakpoints  Table=Kd_table  InterpMethod=Flat  InternalRulePriority=Speed  RndMeth=Simplest
      settings: InputPortMap=u0,u1,u2
  Gain Scheduling Kp : Lookup_n-D  NumberOfTableDimensions=3  BreakpointsForDimension1=ml_breakpoints  BreakpointsForDimension2=l_breakpoints  BreakpointsForDimension3=at_breakpoints  BreakpointsForDimension4=at_breakpoints  Table=Kp_table  InterpMethod=Flat  InternalRulePriority=Speed  RndMeth=Simplest
      settings: InputPortMap=u0,u1,u2
  Gain1 : Gain  Gain=1/T_s2
  Product1 : Product
  Product7 : Product
  Scope1 : Scope  NumInputPorts=2
  Sum1 : Sum  Inputs=|-+
  Sum11 : Sum  Inputs=|++
  Sum2 : Sum  Inputs=-+|
  To Workspace10 : ToWorkspace  VariableName=tita_ref  SaveFormat=Timeseries  SampleTime=-1
      settings: Save2DSignal=2-D array (concatenate along first dimension)
  Zero-Order Hold : ZeroOrderHold  SampleTime=T_s2
  vel_bal* : Outport
  wires:
  Sum2/1 -> Gain1/1
  Gain Scheduling Kd/1 -> Product7/2  "Kd"
  Gain/1 -> Atan/1
  Gain Scheduling Kp/1 -> Product1/1  "Kp"
  theta/1 -> Sum1/1, Scope1/1  "theta"
  Atan/1 -> To Workspace10/1, Scope1/2, Sum1/2  "ref"
  ddx_t_ref/1 -> Gain/1
  Sum1/1 -> Zero-Order Hold/1, Product1/2  "e_tita"
  Sum11/1 -> vel_bal*/1  "vel_bal"
  ml/1 -> Gain Scheduling Kd/1, Gain Scheduling Kp/1
  l_h/1 -> Gain Scheduling Kd/2, Gain Scheduling Kp/2
  ddx_t/1 -> Gain Scheduling Kd/3, Gain Scheduling Kp/3
  Product1/1 -> Sum11/1
  Product7/1 -> Sum11/2
  Zero-Order Hold/1 -> Delay/1, Sum2/2
  Delay/1 -> Sum2/1
  Gain1/1 -> Product7/1

== system PLANTA_COMPLETA/Nivel 2 - Control Regulatorio + Obs/Controlador de izaje ==
  dl_href : Inport
  dl_h : Inport  Port=2
  Discrete-Time Integrator : DiscreteIntegrator  SampleTime=T_s2  ICPrevOutput=DiscIntNeverNeededParam  ICPrevScaledInput=DiscIntNeverNeededParam
  Discrete-Time Integrator1 : DiscreteIntegrator  SampleTime=T_s2  ICPrevOutput=DiscIntNeverNeededParam  ICPrevScaledInput=DiscIntNeverNeededParam
  Gain1 : Gain  Gain=K_hsia
  Gain2 : Gain  Gain=b_ha
  Gain8 : Gain  Gain=K_hsa
  Sum : Sum  Inputs=|+-
  Sum5 : Sum  Inputs=+|+|+
  T_hm* : Outport
  wires:
  Gain2/1 -> Sum5/3
  dl_h/1 -> Sum/2
  Sum5/1 -> T_hm*/1
  dl_href/1 -> Sum/1
  Gain1/1 -> Sum5/1
  Sum/1 -> Gain2/1, Discrete-Time Integrator/1  "d_ek"
  Gain8/1 -> Sum5/2
  Discrete-Time Integrator/1 -> Gain8/1, Discrete-Time Integrator1/1
  Discrete-Time Integrator1/1 -> Gain1/1

== system PLANTA_COMPLETA/Nivel 2 - Control Regulatorio + Obs/Controlador del carro ==
  dx_td : Inport
  dx_t_consig : Inport  Port=2
  Gain : Gain  Gain=T_s2/2
  Gain1 : Gain  Gain=b_ta
  Gain2 : Gain  Gain=K_tsa
  Gain3 : Gain  Gain=T_s2/2
  Gain4 : Gain  Gain=K_tsia
  Scope : Scope
  Scope1 : Scope
  Sum : Sum  Inputs=|+-
  Sum1 : Sum  Inputs=|+-
  Sum2 : Sum  Inputs=|++
  Sum3 : Sum  Inputs=|+-
  Sum4 : Sum  Inputs=|++
  Sum5 : Sum  Inputs=+|+|+
  Unit Delay{,1..3} (4 alike) : UnitDelay  SampleTime=T_s2  HasFrameUpgradeWarning=on
  T_tm* : Outport
  wires:
  Unit Delay3/1 -> Sum4/2  "Ik-1"
  Unit Delay2/1 -> Sum3/2  "ek-1"
  Sum/1 -> Gain1/1, Unit Delay/1, Sum1/1  "d_ek"
  dx_t_consig/1 -> Sum/1
  Gain3/1 -> Sum4/1  "Ik"
  Sum5/1 -> T_tm*/1
  dx_td/1 -> Sum/2
  Sum1/1 -> Gain/1
  Unit Delay/1 -> Sum1/2  "d_ek-1"
  Sum2/1 -> Unit Delay1/1, Sum3/1, Unit Delay2/1, Scope/1, Gain2/1  "ek"
  Gain/1 -> Sum2/1  "Ik"
  Gain2/1 -> Sum5/2
  Sum3/1 -> Gain3/1
  Unit Delay1/1 -> Sum2/2  "Ik-1"
  Sum4/1 -> Gain4/1, Unit Delay3/1
  Gain1/1 -> Sum5/3
  Gain4/1 -> Scope1/1, Sum5/1

== system PLANTA_COMPLETA/Nivel 2 - Control Regulatorio + Obs/Controlador del carro1 ==
  dx_td : Inport
  dx_t_consig : Inport  Port=2
  Discrete-Time Integrator : DiscreteIntegrator  SampleTime=T_s2  ICPrevOutput=DiscIntNeverNeededParam  ICPrevScaledInput=DiscIntNeverNeededParam
  Discrete-Time Integrator1 : DiscreteIntegrator  SampleTime=T_s2  ICPrevOutput=DiscIntNeverNeededParam  ICPrevScaledInput=DiscIntNeverNeededParam
  Gain1 : Gain  Gain=b_ta
  Gain2 : Gain  Gain=K_tsa
  Gain4 : Gain  Gain=K_tsia
  Sum : Sum  Inputs=|+-
  Sum5 : Sum  Inputs=+|+|+
  T_tm* : Outport
  wires:
  Sum/1 -> Gain1/1, Discrete-Time Integrator/1  "d_ek"
  dx_t_consig/1 -> Sum/1
  Sum5/1 -> T_tm*/1
  dx_td/1 -> Sum/2
  Gain2/1 -> Sum5/2
  Gain1/1 -> Sum5/3
  Gain4/1 -> Sum5/1
  Discrete-Time Integrator/1 -> Gain2/1, Discrete-Time Integrator1/1
  Discrete-Time Integrator1/1 -> Gain4/1

== system PLANTA_COMPLETA/Nivel 2 - Control Regulatorio + Obs/Modulador de torque Motor - Izaje ==
  T_hm* : Inport
  First Order Hold : FirstOrderHold  ErrorTolerance=inf
  Gain : Gain  Gain=1/tauhm
  Gain1 : Gain  Gain=1/tauhm
  Integrator : Integrator
  Sum : Sum  Inputs=|+-
  T_hm : Outport
  wires:
  Sum/1 -> Integrator/1
  Integrator/1 -> T_hm/1, Gain1/1
  Gain1/1 -> Sum/2
  First Order Hold/1 -> Gain/1
  Gain/1 -> Sum/1
  T_hm*/1 -> First Order Hold/1

== system PLANTA_COMPLETA/Nivel 2 - Control Regulatorio + Obs/Modulador torque Motor - Carro ==
  T_tm* : Inport
  First Order Hold : FirstOrderHold  ErrorTolerance=inf
  Gain : Gain  Gain=1/tautm
  Gain1 : Gain  Gain=1/tautm
  Integrator : Integrator
  Sum : Sum  Inputs=|+-
  T_tm : Outport
  wires:
  Integrator/1 -> Gain1/1, T_tm/1
  T_tm*/1 -> First Order Hold/1
  First Order Hold/1 -> Gain/1
  Gain/1 -> Sum/1
  Sum/1 -> Integrator/1
  Gain1/1 -> Sum/2

== system PLANTA_COMPLETA/Nivel 2 - Control Regulatorio + Obs/Observador_Control_Posicion ==
  T_tm* : Inport
  x_td_real : Inport  Port=2
  x_t_ref : Inport  Port=3
  theta_l : Inport  Port=4
  F_hw : Inport  Port=5
  Discrete Derivative : simulink/Discrete/Discrete Derivative  gainval=1.0  ICPrevScaledInput=0.0  OutMin=[]  OutMax=[]  OutDataType=fixdt(1, 16)  OutScaling=2^-10  DoSatur=off
  Fuerzas de tension de cable en Carro : Subsystem
  Observador : Subsystem
  Subsystem : Subsystem
  Traslacion del carro : Subsystem
  ddx_t : Outport
  dx_t_pos : Outport  Port=2
  dx_td_obs : Outport  Port=3
  wires:
  Observador/1(dx_td_obs) -> Fuerzas de tension de cable en Carro/2(dx_td), dx_td_obs/1  "dx_td_obs"
  x_td_real/1 -> Fuerzas de tension de cable en Carro/1(x_td), Observador/1(x_td)
  x_t_ref/1 -> Subsystem/2(xt_ref)
  Subsystem/1(dxt_pos) -> dx_t_pos/1
  Traslacion del carro/1(x_t) -> Fuerzas de tension de cable en Carro/3(x_t), Subsystem/1(xt_obs)  "x_t_obs"
  Traslacion del carro/2(dx_t) -> Fuerzas de tension de cable en Carro/4(dx_t), Discrete Derivative/1  "dx_t_obs"
  theta_l/1 -> Traslacion del carro/3(theta_l)
  F_hw/1 -> Traslacion del carro/2(F_hw)
  Fuerzas de tension de cable en Carro/1(F_tw) -> Traslacion del carro/1(F_tw)
  T_tm*/1 -> Observador/2(T_tm*)
  Discrete Derivative/1 -> ddx_t/1

== system PLANTA_COMPLETA/PLANTA/ACC DE CARRO ==
  F_tw : Inport
  BRK_t : Inport  Port=2
  T_tm : Inport  Port=3
  Freno : Subsystem
  Gain : Gain  Gain=rtd
  Gain1 : Gain  Gain=it
  Gain2 : Gain  Gain=(btm*(it)^2+btd)/rtd
  Gain3 : Gain  Gain=rtd/(Jtd+Jtm_tb*(it)^2)
  Integrator : Integrator  InitialCondition=dx_td_ini
  Integrator1 : Integrator  InitialCondition=x_td_ini
  Sum : Sum  Inputs=|++
  Sum1 : Sum  Inputs=-|+|-
  x_td : Outport
  dx_td : Outport  Port=2
  wires:
  T_tm/1 -> Sum/2
  Gain/1 -> Sum1/1
  Gain3/1 -> Integrator/1  "ddx_td"
  Sum1/1 -> Gain3/1
  F_tw/1 -> Gain/1
  Gain1/1 -> Sum1/2
  Integrator1/1 -> x_td/1
  Gain2/1 -> Sum1/3
  Sum/1 -> Gain1/1
  BRK_t/1 -> Freno/2(BRK_t)
  Freno/1(T_tb) -> Sum/1
  Integrator/1 -> dx_td/1, Freno/1(dx_td), Integrator1/1, Gain2/1

== system PLANTA_COMPLETA/PLANTA/ACC DE IZAJE ==
  T_hm : Inport
  F_hw : Inport  Port=2
  BRK_h : Inport  Port=3
  BRK_hE : Inport  Port=4
  Add : Sum  Inputs=+++-
  Freno : Subsystem
  Freno Emergencia : Subsystem
  Gain : Gain  Gain=rhd
  Gain1 : Gain  Gain=ih
  Gain2 : Gain  Gain=(2*bhd+2*bhm*(ih)^2)/rhd
  Gain3 : Gain  Gain=-2/rhd
  Gain4 : Gain  Gain=ih
  Gain6 : Gain  Gain=-rhd/(2*Jhd_hEb+2*Jhm_hb*(ih)^2)
  Integrator : Integrator  InitialCondition=l_h_ini
  Integrator1 : Integrator  InitialCondition=dl_h_ini
  Sum : Sum  Inputs=-|+||
  l_h : Outport
  dl_h : Outport  Port=2
  wires:
  Gain1/1 -> Add/2
  Integrator1/1 -> Gain2/1, Gain3/1, Integrator/1, dl_h/1
  F_hw/1 -> Gain/1
  T_hm/1 -> Sum/2
  Freno Emergencia/1(T_hEB) -> Add/3
  BRK_hE/1 -> Freno Emergencia/2(BRK_hE)
  Gain4/1 -> Freno/1(w_hm)  "w_hm"
  Gain/1 -> Add/4
  Integrator/1 -> l_h/1
  Gain3/1 -> Freno Emergencia/1(w_hd), Gain4/1  "w_hd"
  Sum/1 -> Gain1/1
  Add/1 -> Gain6/1
  Freno/1(T_hb) -> Sum/1
  Gain2/1 -> Add/1
  BRK_h/1 -> Freno/2(BRK_h)
  Gain6/1 -> Integrator1/1  "ddl_h"

== system PLANTA_COMPLETA/PLANTA/Altura perfil obstaculos (A partir de posicion x_l) ==
  x_l : Inport
  Ajuste referencia : Constant  Value=30
  Calculo : MATLAB Function  TreatAsAtomicUnit=on
  Data Store Read : DataStoreRead  DataStoreName=y0_global  IndexOptions=Index vector (dialog)  Indices=1  OutputSizes=1
  Data Type Conversion : DataTypeConversion  OutDataTypeStr=int32  RndMeth=Ceiling  SaturateOnIntegerOverflow=off
  Gain1 : Gain  Gain=1/Wc
  Sum : Sum  Inputs=|++
  yc0_xl : Outport
  wires:
  Data Store Read/1 -> Calculo/1(y0_array)
  Gain1/1 -> Data Type Conversion/1
  Ajuste referencia/1 -> Sum/2
  Sum/1 -> Gain1/1
  x_l/1 -> Sum/1
  Calculo/1(yc0_xt) -> yc0_xl/1
  Data Type Conversion/1 -> Calculo/2(index)

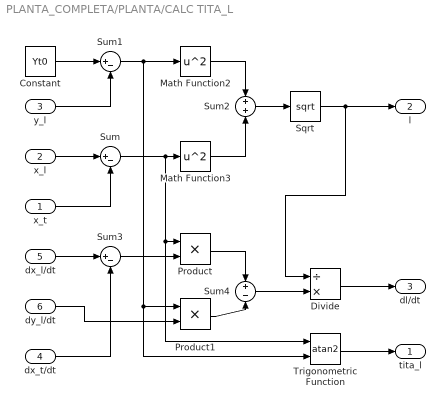
== system PLANTA_COMPLETA/PLANTA/CALC TITA_L ==
  x_t : Inport
  x_l : Inport  Port=2
  y_l : Inport  Port=3
  dx_t/dt : Inport  Port=4
  dx_l/dt : Inport  Port=5
  dy_l/dt : Inport  Port=6
  Constant : Constant  Value=Yt0
  Divide : Product  Inputs=/*
  Math Function2 : Math  Operator=square
  Math Function3 : Math  Operator=square
  Product : Product
  Product1 : Product
  Sqrt : Sqrt
  Sum : Sum  Inputs=|+-
  Sum1 : Sum  Inputs=|+-
  Sum2 : Sum  Inputs=+|+
  Sum3 : Sum  Inputs=|+-
  Sum4 : Sum  Inputs=+|-
  Trigonometric Function : Trigonometry  Operator=atan2
  tita_l : Outport
  l : Outport  Port=2
  dl/dt : Outport  Port=3
  wires:
  Product/1 -> Sum4/1
  Product1/1 -> Sum4/2
  x_l/1 -> Sum/1
  dx_t/dt/1 -> Sum3/2
  y_l/1 -> Sum1/2
  Sum/1 -> Product/1, Trigonometric Function/1, Math Function3/1
  Sqrt/1 -> l/1, Divide/1
  Sum2/1 -> Sqrt/1
  Sum4/1 -> Divide/2
  Sum1/1 -> Product1/1, Trigonometric Function/2, Math Function2/1
  Math Function2/1 -> Sum2/1
  dx_l/dt/1 -> Sum3/1
  x_t/1 -> Sum/2
  Constant/1 -> Sum1/1
  Sum3/1 -> Product/2
  dy_l/dt/1 -> Product1/2
  Math Function3/1 -> Sum2/2
  Trigonometric Function/1 -> tita_l/1
  Divide/1 -> dl/dt/1

== system PLANTA_COMPLETA/PLANTA/FIN_CARRERA_IZAJE ==
  l_h : Inport
  Constant : Constant  Value=Yt0
  Constant1 : Constant  Value=-19.5
  Constant2 : Constant  Value=-20
  Constant3 : Constant  Value=49.5
  Constant4 : Constant  Value=50
  Relational Operator : RelationalOperator  Operator=<=  OutDataTypeStr=boolean  RndMeth=Simplest  InputSameDT=off
  Relational Operator1 : RelationalOperator  Operator=<=  OutDataTypeStr=boolean  RndMeth=Simplest  InputSameDT=off
  Relational Operator2 : RelationalOperator  OutDataTypeStr=boolean  RndMeth=Simplest  InputSameDT=off
  Relational Operator3 : RelationalOperator  OutDataTypeStr=boolean  RndMeth=Simplest  InputSameDT=off
  Sum : Sum  Inputs=|-+
  FC_INF : Outport
  FCE_INF : Outport  Port=2
  FC_SUP : Outport  Port=3
  FCE_SUP : Outport  Port=4
  wires:
  Sum/1 -> Relational Operator3/1, Relational Operator2/1, Relational Operator/1, Relational Operator1/1  "y_h"
  Relational Operator3/1 -> FCE_SUP/1
  Constant4/1 -> Relational Operator3/2
  Relational Operator2/1 -> FC_SUP/1
  Constant3/1 -> Relational Operator2/2
  Constant1/1 -> Relational Operator/2
  Constant2/1 -> Relational Operator1/2
  Relational Operator/1 -> FC_INF/1
  Constant/1 -> Sum/2
  Relational Operator1/1 -> FCE_INF/1
  l_h/1 -> Sum/1

== system PLANTA_COMPLETA/PLANTA/Fin de carrera Carro ==
  x_t : Inport
  Constant : Constant  Value=-29.5
  Constant1 : Constant  Value=-30
  Constant2 : Constant  Value=49.5
  Constant3 : Constant  Value=50
  Relational Operator : RelationalOperator  Operator=<=  OutDataTypeStr=boolean  RndMeth=Simplest  InputSameDT=off
  Relational Operator1 : RelationalOperator  Operator=<=  OutDataTypeStr=boolean  RndMeth=Simplest  InputSameDT=off
  Relational Operator2 : RelationalOperator  OutDataTypeStr=boolean  RndMeth=Simplest  InputSameDT=off
  Relational Operator3 : RelationalOperator  OutDataTypeStr=boolean  RndMeth=Simplest  InputSameDT=off
  FC_IZQ : Outport
  FCE_IZQ : Outport  Port=2
  FC_DER : Outport  Port=3
  FCE_DER : Outport  Port=4
  wires:
  Relational Operator/1 -> FC_IZQ/1
  Constant1/1 -> Relational Operator1/2
  Relational Operator1/1 -> FCE_IZQ/1
  Constant2/1 -> Relational Operator2/2
  Relational Operator2/1 -> FC_DER/1
  Relational Operator3/1 -> FCE_DER/1
  Constant3/1 -> Relational Operator3/2
  Constant/1 -> Relational Operator/2
  x_t/1 -> Relational Operator2/1, Relational Operator3/1, Relational Operator/1, Relational Operator1/1

== system PLANTA_COMPLETA/PLANTA/Masa de contenedor (A partir de posicion x_l) ==
  TLK : Inport
  x_l : Inport  Port=2
  masas_array : Inport  Port=3
  Ajuste referencia : Constant  Value=30
  Calculo : MATLAB Function  TreatAsAtomicUnit=on
  Constant : Constant  Value=0
  Data Type Conversion : DataTypeConversion  OutDataTypeStr=int32  RndMeth=Ceiling  SaturateOnIntegerOverflow=off
  Edge Detector : spsEdgeDetectorLib/Edge Detector  model=Falling  ic=0  Ts=-1
  Edge Detector1 : spsEdgeDetectorLib/Edge Detector  model=Rising  ic=0  Ts=-1
  Gain1 : Gain  Gain=1/Wc
  S-R Flip-Flop : simulink_extras/Flip Flops/S-R Flip-Flop  initial_condition=0
  Sample and Hold : dspsigops/Sample and Hold  trig=Rising edge  initCond=0  latchinput=off
  Sum : Sum  Inputs=|++
  Switch : Switch  Criteria=u2 ~= 0  SaturateOnIntegerOverflow=off  InputSameDT=off
  Unit Delay : UnitDelay  SampleTime=-1  HasFrameUpgradeWarning=on
  Mc_X : Outport
  wires:
  Data Type Conversion/1 -> Calculo/2(index)
  Gain1/1 -> Data Type Conversion/1
  Ajuste referencia/1 -> Sum/2
  Sum/1 -> Gain1/1
  x_l/1 -> Sum/1
  TLK/1 -> Unit Delay/1
  Edge Detector/1 -> S-R Flip-Flop/2
  Edge Detector1/1 -> S-R Flip-Flop/1
  Sample and Hold/1 -> Switch/1
  Unit Delay/1 -> Edge Detector1/1, Edge Detector/1
  Calculo/1(Mc_X) -> Sample and Hold/1
  masas_array/1 -> Calculo/1(masas_array)
  Constant/1 -> Switch/3
  S-R Flip-Flop/1 -> Switch/2, Sample and Hold/Trigger
  Switch/1 -> Mc_X/1

== system PLANTA_COMPLETA/PLANTA/PERFIL_OBSTACULOS ==
  note: LIDAR
  x_t : Inport
  Ajuste distancia LIDAR : dspsigops/Variable Fractional Delay  mode=OBSOLETE  modeActive=Linear  L=4  FarrowL=4  R=10  alpha=1  dmax=100  InputProcessing=Columns as channels (frame based)  ic=0  noDFT=off  fallbackFIR=Clip to the minimum value necessary for centered kernel  fallbackFarrow=Clip to the minimum value necessary for centered kernel  roundingMode=Zero  overflowMode=off
  Ajuste referencia : Constant  Value=30
  Constant : Constant  Value=Yt0
  Data Type Conversion : DataTypeConversion  OutDataTypeStr=int32  RndMeth=Ceiling  SaturateOnIntegerOverflow=off
  Delay : Delay  DelayLength=1  InputProcessing=Columns as channels (frame based)  SampleTime=0.001
  Delay espacial : Constant  Value=3/Wc
  Gain : Gain  Gain=1/Wc
  Perfil obstaculos (ENTORNO) : FromWorkspace  VariableName=y0
  Posicion LIDAR : Constant  Value=3
  Sum : Sum  Inputs=|++
  Sum1 : Sum  Inputs=|++
  Sum2 : Sum  Inputs=+-|
  sensor : MATLAB Function  TreatAsAtomicUnit=on
  yc0_xt : Outport
  wires:
  Delay/1 -> Sum1/1
  Sum/1 -> Gain/1
  Constant/1 -> Sum2/1
  Sum2/1 -> yc0_xt/1
  Sum1/1 -> Sum/1
  Delay espacial/1 -> Ajuste distancia LIDAR/2
  Ajuste distancia LIDAR/1 -> Sum2/2
  Data Type Conversion/1 -> sensor/2(index)
  Perfil obstaculos (ENTORNO)/1 -> sensor/1(y0_array)
  sensor/1(distancia) -> Ajuste distancia LIDAR/1
  Posicion LIDAR/1 -> Sum1/2
  Gain/1 -> Data Type Conversion/1
  x_t/1 -> Delay/1
  Ajuste referencia/1 -> Sum/2

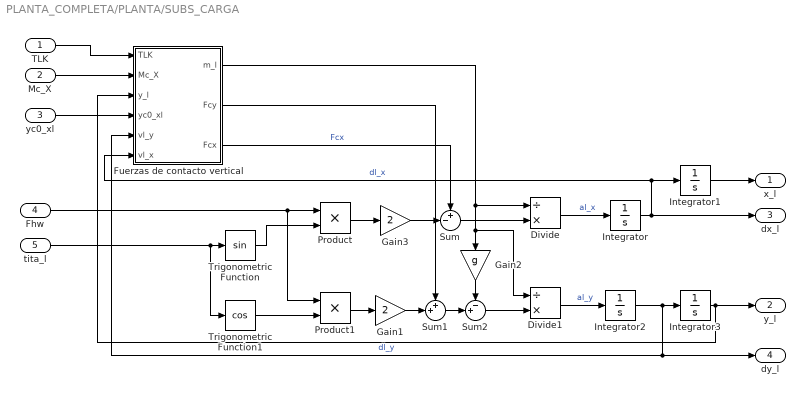
== system PLANTA_COMPLETA/PLANTA/SUBS_CARGA ==
  TLK : Inport
  Mc_X : Inport  Port=2
  yc0_xl : Inport  Port=3
  Fhw : Inport  Port=4
  tita_l : Inport  Port=5
  Divide : Product  Inputs=/*
  Divide1 : Product  Inputs=/*
  Fuerzas de contacto vertical : Subsystem
  Gain1 : Gain  Gain=2
  Gain2 : Gain  Gain=g
  Gain3 : Gain  Gain=2
  Integrator : Integrator  InitialCondition=dx_l_ini
  Integrator1 : Integrator  InitialCondition=x_l_ini
  Integrator2 : Integrator  InitialCondition=dy_l_ini
  Integrator3 : Integrator  InitialCondition=y_l_ini
  Product : Product
  Product1 : Product
  Sum : Sum  Inputs=+-|
  Sum1 : Sum  Inputs=++|
  Sum2 : Sum  Inputs=-+|
  Trigonometric Function : Trigonometry
  Trigonometric Function1 : Trigonometry  Operator=cos
  x_l : Outport
  y_l : Outport  Port=2
  dx_l : Outport  Port=3
  dy_l : Outport  Port=4
  wires:
  Divide1/1 -> Integrator2/1  "al_y"
  Sum2/1 -> Divide1/2
  Integrator2/1 -> dy_l/1, Fuerzas de contacto vertical/5(vl_y), Integrator3/1  "dl_y"
  Fhw/1 -> Product/1, Product1/1
  Divide/1 -> Integrator/1  "al_x"
  Product1/1 -> Gain1/1
  Sum/1 -> Divide/2
  Fuerzas de contacto vertical/1(m_l) -> Divide/1, Divide1/1, Gain2/1
  Gain1/1 -> Sum1/2
  Trigonometric Function1/1 -> Product1/2
  Fuerzas de contacto vertical/3(Fcx) -> Sum/1  "Fcx"
  Gain2/1 -> Sum2/1
  Integrator/1 -> Fuerzas de contacto vertical/6(vl_x), Integrator1/1, dx_l/1  "dl_x"
  Product/1 -> Gain3/1
  yc0_xl/1 -> Fuerzas de contacto vertical/4(yc0_xl)
  Trigonometric Function/1 -> Product/2
  Integrator1/1 -> x_l/1
  Sum1/1 -> Sum2/2
  Gain3/1 -> Sum/2
  Mc_X/1 -> Fuerzas de contacto vertical/2(Mc_X)
  TLK/1 -> Fuerzas de contacto vertical/1(TLK)
  Fuerzas de contacto vertical/2(Fcy) -> Sum1/1
  Integrator3/1 -> Fuerzas de contacto vertical/3(y_l), y_l/1
  tita_l/1 -> Trigonometric Function1/1, Trigonometric Function/1

== system PLANTA_COMPLETA/PLANTA/TENSION CABLE CARRO ==
  x_td : Inport
  dx_td : Inport  Port=2
  x_t : Inport  Port=3
  dx_t : Inport  Port=4
  Add : Sum  Inputs=+-
  Add1 : Sum  Inputs=+-
  Add2 : Sum
  Gain : Gain  Gain=Ktw
  Gain1 : Gain  Gain=btw
  F_tw : Outport
  wires:
  Add1/1 -> Gain1/1
  Add/1 -> Gain/1
  Gain1/1 -> Add2/2
  x_td/1 -> Add/1
  dx_t/1 -> Add1/2
  dx_td/1 -> Add1/1
  Gain/1 -> Add2/1
  Add2/1 -> F_tw/1
  x_t/1 -> Add/2

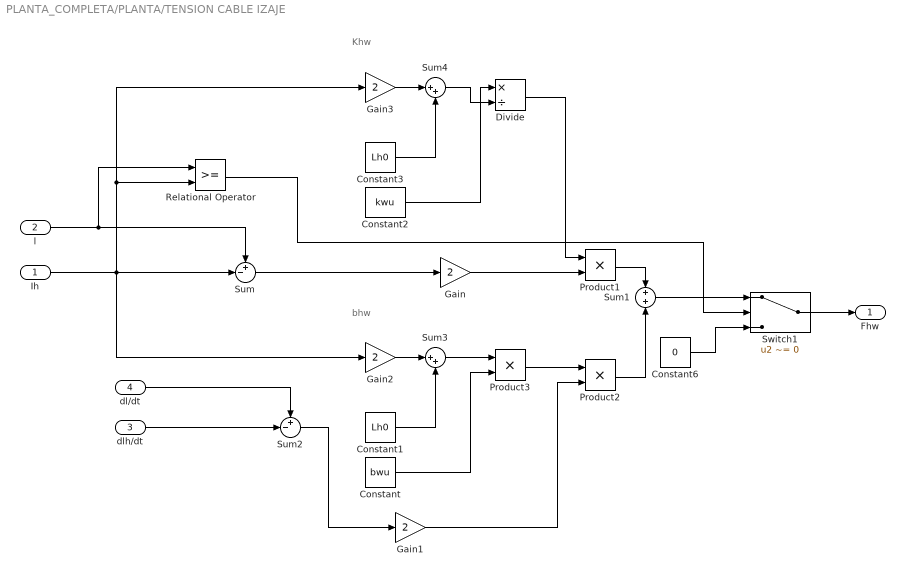
== system PLANTA_COMPLETA/PLANTA/TENSION CABLE IZAJE ==
  note: Khw
  note: bhw
  Ih : Inport
  l : Inport  Port=2
  dlh/dt : Inport  Port=3
  dl/dt : Inport  Port=4
  Constant : Constant  Value=bwu
  Constant1 : Constant  Value=Lh0
  Constant2 : Constant  Value=kwu
  Constant3 : Constant  Value=Lh0
  Constant6 : Constant  Value=0  OutDataTypeStr=double
  Divide : Product  Inputs=*/
  Gain : Gain  Gain=2
  Gain1 : Gain  Gain=2
  Gain2 : Gain  Gain=2  OutDataTypeStr=Inherit: Inherit via back propagation
  Gain3 : Gain  Gain=2  OutDataTypeStr=Inherit: Inherit via back propagation
  Product1 : Product
  Product2 : Product
  Product3 : Product
  Relational Operator : RelationalOperator  OutDataTypeStr=boolean  RndMeth=Simplest  InputSameDT=off
  Sum : Sum  Inputs=+-|
  Sum1 : Sum  Inputs=+|+
  Sum2 : Sum  Inputs=+-|
  Sum3 : Sum  Inputs=|++
  Sum4 : Sum  Inputs=|++
  Switch1 : Switch  Criteria=u2 ~= 0  SaturateOnIntegerOverflow=off  InputSameDT=off
  Fhw : Outport
  wires:
  l/1 -> Sum/1, Relational Operator/1
  dlh/dt/1 -> Sum2/2
  Sum/1 -> Gain/1
  Product2/1 -> Sum1/2
  Sum1/1 -> Switch1/1
  Gain/1 -> Product1/2
  Product3/1 -> Product2/1
  Sum4/1 -> Divide/2
  Sum2/1 -> Gain1/1
  Divide/1 -> Product1/1
  Product1/1 -> Sum1/1
  dl/dt/1 -> Sum2/1
  Constant/1 -> Product3/2
  Sum3/1 -> Product3/1
  Gain3/1 -> Sum4/1
  Ih/1 -> Gain2/1, Sum/2, Gain3/1, Relational Operator/2
  Constant1/1 -> Sum3/2
  Constant3/1 -> Sum4/2
  Relational Operator/1 -> Switch1/2
  Constant2/1 -> Divide/1
  Gain1/1 -> Product2/2
  Gain2/1 -> Sum3/1
  Constant6/1 -> Switch1/3
  Switch1/1 -> Fhw/1

== system PLANTA_COMPLETA/PLANTA/TRASLAC CARRO ==
  F_tw : Inport
  F_hw : Inport  Port=2
  theta_l : Inport  Port=3
  Gain : Gain  Gain=2
  Gain1 : Gain  Gain=bt
  Gain2 : Gain  Gain=1/Mt
  Integrator : Integrator  InitialCondition=dx_t_ini
  Integrator1 : Integrator  InitialCondition=x_t_ini
  Product : Product
  Sin : Trigonometry
  Sum : Sum  Inputs=++-
  x_t : Outport
  dx_t : Outport  Port=2
  wires:
  Gain1/1 -> Sum/3
  Integrator1/1 -> x_t/1
  theta_l/1 -> Sin/1
  Sin/1 -> Product/2
  Sum/1 -> Gain2/1
  F_tw/1 -> Sum/1
  F_hw/1 -> Product/1
  Gain/1 -> Sum/2
  Integrator/1 -> dx_t/1, Gain1/1, Integrator1/1
  Product/1 -> Gain/1
  Gain2/1 -> Integrator/1  "ddx_t"
